simulink model "upqc"  (R2021a)
settings: Solver=VariableStepAuto  StartTime=0.0  StopTime=0.5  RelTol=1e-3
libraries: spsDiodeLib x18, spsSeriesRLCBranchLib x16, spsIGBTLib x6, spsCurrentMeasurementLib x5, spsGroundLib x3, spsThreePhaseSeriesRLCBranchLib x3, spsVoltageMeasurementLib x3, spsThreePhaseProgrammableVoltageSourceLib x3, spsThreePhaseVIMeasurementLib x3, spsPVArrayLib x1, spspowerguiLib x1
settings Model: Creator=Dell  LastModifiedBy=Dell

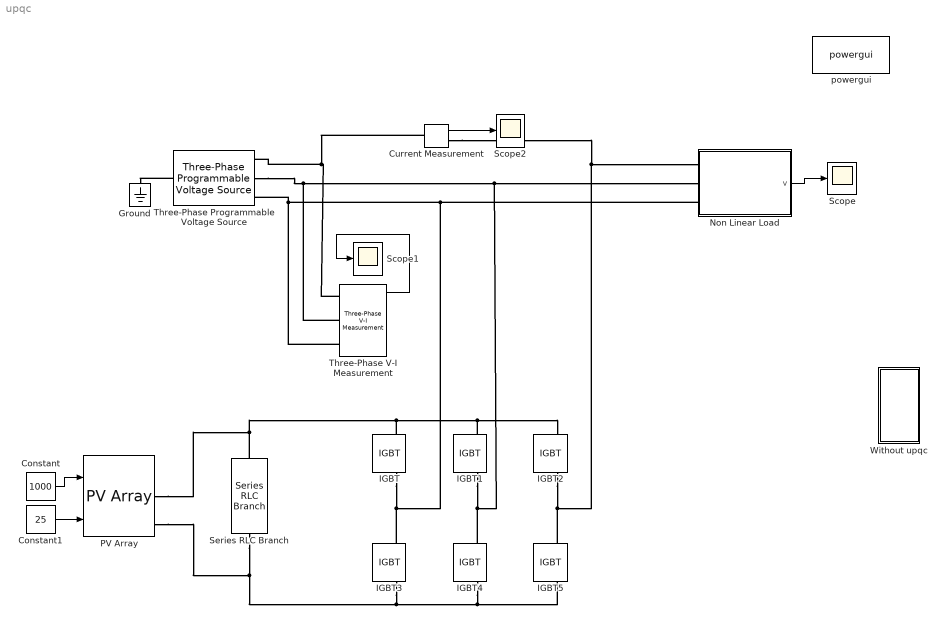
== system upqc ==
  Constant : Constant  Value=1000
  Constant1 : Constant  Value=25
  Current Measurement : spsCurrentMeasurementLib/Current Measurement  PhasorSimulation=off  OutputType=Complex  PSBequivalent=0
  Ground : spsGroundLib/Ground  LConnTagsString=a
  IGBT{,1..5} (6 alike) : spsIGBTLib/IGBT  Ron=0.001  Lon=0  Vf=1  Tf=1e-6  Tt=2e-6  IC=0  Rs=1e5  Cs=inf  Measurements=on
  Non Linear Load : Subsystem
  PV Array : spsPVArrayLib/PV Array  Npar=40  Nser=10  PlotType=array @ 1000 W/m2 & specified temperatures  S_vec="[ 1000  500  100 ]"  Temp_C_vec="[ 45 25  ]"  ModuleName=User-defined  PlotWhenSelected=off  Pm=213.15  Ncell=60  Voc=36.3  Isc=7.84  Vm=29  Im=7.35  beta_Voc_pc=-0.36099  alpha_Isc_pc=0.102  beta_Voc=-0.13104  alpha_Isc=0.0079968  IL=7.8654  I0=2.9273e-10  nI=0.98119  Rsh=313.0553  Rs=0.39381  RobustModel=off  RobustCellTemperature=313.3991  BAL=on  Tc=1e-6  Tfilter=5e-5
  Scope : Scope
  Scope1 : Scope
  Scope2 : Scope
  Series RLC Branch : spsSeriesRLCBranchLib/Series RLC Branch  LConnTagsString=__new0  RConnTagsString=__new0  BranchType=C  Resistance=1  Inductance=1e-3  SetiL0=off  InitialCurrent=0  Capacitance=1e-6  Setx0=off  InitialVoltage=0  Measurements=None
  Three-Phase Programmable Voltage Source : spsThreePhaseProgrammableVoltageSourceLib/Three-Phase Programmable Voltage Source  PositiveSequence="[400  0 50]"  VariationEntity=Amplitude  VariationType=Table of time-amplitude pairs  VariationTypeAlt=Step  VariationStep=0.5  VariationRate=10  VariationMagnitude=0.3  VariationFrequency=2  VariationTiming=[1 2]  VariationPhaseA=off  Amplitudes=[1 0.7 1 1.3 1]  TimeValues=[0 0.9 1 1.6 1.7]  HarmonicGeneration=on  HarmonicA=[5 0.2 -0 2]  HarmonicB=[7 0.05 0 1]  Timing=[0.3 0.4]  BusType=swing  Pref=0  Qref=0  Qmin=-inf  Qmax=inf
  Three-Phase V-I Measurement : spsThreePhaseVIMeasurementLib/Three-Phase V-I Measurement  VoltageMeasurement=phase-to-ground  SetLabelV=off  LabelV=Vabc  Vpu=off  VpuLL=off  CurrentMeasurement=yes  SetLabelI=off  LabelI=Iabc  Ipu=off  Pbase=100e6  Vbase=500e3  OutputType=Complex  PhasorSimulation=off  PSBequivalent=0
  Without upqc : Subsystem
  powergui : spspowerguiLib/powergui  Priority=1  SimulationMode=Continuous  SampleTime=50e-6  frequency=60  Iterations=50  frequencyindice=50  Pbase=100e6  ErrMax=1e-4  UnitsV=kV  UnitsW=MW  buscounter=0  FunctionMessages=off  echomessages=off  EnableUseOfTLC=off  CurrentSourceSwitches=off  DisableSnubberDevices=off  DisableRonSwitches=off  DisableVfSwitches=off  DisplayEquations=off  AutomaticDiscreteSolvers=off  SolverType=Tustin/Backward Euler (TBE)  Interpol=off  ExternalGateDelay=off  methode=off  Ts=100  x0status=blocks  SPID=on  SwTol=0  HookPort=off  NonlinearTolerance=1e-4  nMaxIteration=100  ContinueOnMaxIteration=off  RestoreLinks=warning  ResistiveCurrentMeasurement=off  Frange=[0:2:500]  Ylog=off  Xlog=on  ShowGrid=off  save=off  variable=ZData  structure=0  ZoomFFT=off  StartTime=0.0  cycles=1  DisplayStyle=1  fundamental=60  FreqAxis=off  MaxFrequency=1000  frequencyindicesteady=1  RmsSteady=1  display=off
  wires:
  Three-Phase V-I Measurement/1 -> Scope1/1
  Non Linear Load/1(v) -> Scope/1
  Constant1/1 -> PV Array/2
  Constant/1 -> PV Array/1
  Current Measurement/1 -> Scope2/1
  connections:
  Three-Phase Programmable Voltage Source/LConn1 -- Ground/LConn1
  Three-Phase V-I Measurement/LConn3 -- IGBT/RConn1 -- IGBT3/LConn1 -- Non Linear Load/LConn3 -- Three-Phase Programmable Voltage Source/RConn3
  Three-Phase V-I Measurement/LConn2 -- Three-Phase Programmable Voltage Source/RConn2 -- IGBT1/RConn1 -- IGBT4/LConn1 -- Non Linear Load/LConn2
  IGBT5/LConn1 -- IGBT2/RConn1 -- Current Measurement/RConn1 -- Non Linear Load/LConn1
  IGBT/LConn1 -- PV Array/RConn1 -- Series RLC Branch/LConn1 -- IGBT1/LConn1 -- IGBT2/LConn1
  IGBT3/RConn1 -- Series RLC Branch/RConn1 -- PV Array/RConn2 -- IGBT4/RConn1 -- IGBT5/RConn1
  Three-Phase V-I Measurement/LConn1 -- Current Measurement/LConn1 -- Three-Phase Programmable Voltage Source/RConn1

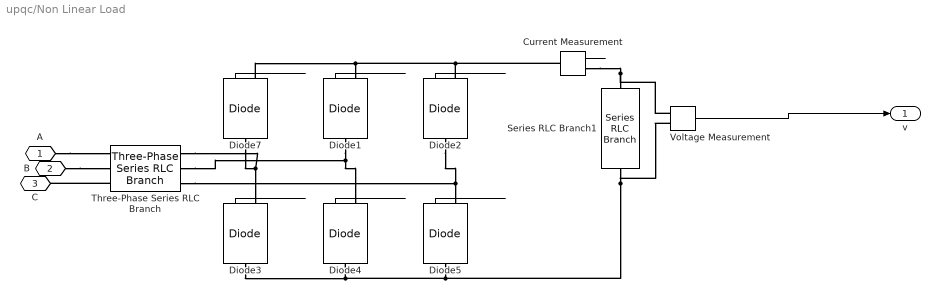
== system upqc/Non Linear Load ==
  Current Measurement : spsCurrentMeasurementLib/Current Measurement  PhasorSimulation=off  OutputType=Complex  PSBequivalent=0
  Diode{1..5,7} (6 alike) : spsDiodeLib/Diode  Ron=0.001  Lon=0  Vf=0.8  IC=0  UseSnubber=0  Rs=500  Cs=250e-9  Measurements=on
  Series RLC Branch1 : spsSeriesRLCBranchLib/Series RLC Branch  LConnTagsString=__new0  RConnTagsString=__new0  BranchType=RL  Resistance=1  Inductance=1e-3  SetiL0=off  InitialCurrent=0  Capacitance=1e-6  Setx0=off  InitialVoltage=0  Measurements=None
  Three-Phase Series RLC Branch : spsThreePhaseSeriesRLCBranchLib/Three-Phase Series RLC Branch  LConnTagsString=A|B|C  RConnTagsString=A|B|C  BranchType=RL  Resistance=1  Inductance=1e-3  Capacitance=1e-6  Measurements=None
  Voltage Measurement : spsVoltageMeasurementLib/Voltage Measurement  PhasorSimulation=off  OutputType=Complex  PSBequivalent=0
  A : PMIOPort  Side=Left
  B : PMIOPort  Port=2  Side=Left
  C : PMIOPort  Port=3  Side=Left
  v : Outport
  wires:
  Diode5/1 -> ?
  Diode2/1 -> ?
  Current Measurement/1 -> ?
  Diode1/1 -> ?
  Diode7/1 -> ?
  Voltage Measurement/1 -> v/1
  Diode4/1 -> ?
  Diode3/1 -> ?
  connections:
  Diode2/LConn1 -- Diode5/RConn1 -- Three-Phase Series RLC Branch/RConn3
  Diode3/LConn1 -- Voltage Measurement/LConn2 -- Series RLC Branch1/RConn1 -- Diode5/LConn1 -- Diode4/LConn1
  Diode1/LConn1 -- Diode4/RConn1 -- Three-Phase Series RLC Branch/RConn2
  Current Measurement/RConn1 -- Voltage Measurement/LConn1 -- Series RLC Branch1/LConn1
  Diode7/RConn1 -- Current Measurement/LConn1 -- Diode2/RConn1 -- Diode1/RConn1
  Diode7/LConn1 -- Diode3/RConn1 -- Three-Phase Series RLC Branch/RConn1
  Three-Phase Series RLC Branch/LConn3 -- C/RConn1
  A/RConn1 -- Three-Phase Series RLC Branch/LConn1
  B/RConn1 -- Three-Phase Series RLC Branch/LConn2

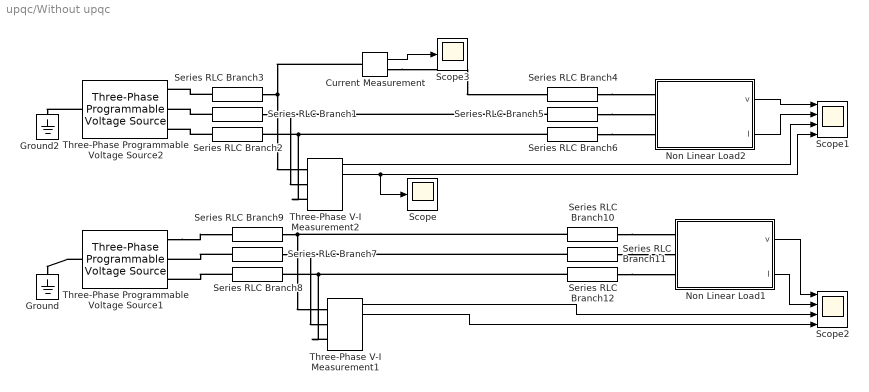
== system upqc/Without upqc ==
  Current Measurement : spsCurrentMeasurementLib/Current Measurement  PhasorSimulation=off  OutputType=Complex  PSBequivalent=0
  Ground : spsGroundLib/Ground  LConnTagsString=a
  Ground2 : spsGroundLib/Ground  LConnTagsString=a
  Non Linear Load1 : Subsystem
  Non Linear Load2 : Subsystem
  Scope : Scope
  Scope1 : Scope  NumInputPorts=4
  Scope2 : Scope  NumInputPorts=4
  Scope3 : Scope
  Series RLC Branch{1..12} (12 alike) : spsSeriesRLCBranchLib/Series RLC Branch  LConnTagsString=__new0  RConnTagsString=__new0  BranchType=RL  Resistance=2000  Inductance=1e-3  SetiL0=off  InitialCurrent=0  Capacitance=1e-6  Setx0=off  InitialVoltage=0  Measurements=None
  Three-Phase Programmable Voltage Source1 : spsThreePhaseProgrammableVoltageSourceLib/Three-Phase Programmable Voltage Source  PositiveSequence="[400  0 50]"  VariationEntity=Amplitude  VariationType=Table of time-amplitude pairs  VariationTypeAlt=Step  VariationStep=0.5  VariationRate=10  VariationMagnitude=0.3  VariationFrequency=2  VariationTiming=[1 2]  VariationPhaseA=off  Amplitudes=[1 0.7 1 1.3 1]  TimeValues=[0 0.9 1 1.6 1.7]  HarmonicGeneration=on  HarmonicA=[5 0.2 -0 2]  HarmonicB=[7 0.05 0 1]  Timing=[0.3 0.4]  BusType=swing  Pref=0  Qref=0  Qmin=-inf  Qmax=inf
  Three-Phase Programmable Voltage Source2 : spsThreePhaseProgrammableVoltageSourceLib/Three-Phase Programmable Voltage Source  PositiveSequence="[400  0 50]"  VariationEntity=None  VariationType=Table of time-amplitude pairs  VariationTypeAlt=Step  VariationStep=0.5  VariationRate=10  VariationMagnitude=0.3  VariationFrequency=2  VariationTiming=[1 2]  VariationPhaseA=off  Amplitudes=[1 0.7 1 1.3 1]  TimeValues=[0 0.9 1 1.6 1.7]  HarmonicGeneration=off  HarmonicA=[5 0.2 -0 2]  HarmonicB=[7 0.05 0 1]  Timing=[0.3 0.4]  BusType=swing  Pref=0  Qref=0  Qmin=-inf  Qmax=inf
  Three-Phase V-I Measurement1 : spsThreePhaseVIMeasurementLib/Three-Phase V-I Measurement  VoltageMeasurement=phase-to-ground  SetLabelV=off  LabelV=Vabc  Vpu=off  VpuLL=off  CurrentMeasurement=yes  SetLabelI=off  LabelI=Iabc  Ipu=off  Pbase=100e6  Vbase=500e3  OutputType=Complex  PhasorSimulation=off  PSBequivalent=0
  Three-Phase V-I Measurement2 : spsThreePhaseVIMeasurementLib/Three-Phase V-I Measurement  VoltageMeasurement=phase-to-ground  SetLabelV=off  LabelV=Vabc  Vpu=off  VpuLL=off  CurrentMeasurement=yes  SetLabelI=off  LabelI=Iabc  Ipu=off  Pbase=100e6  Vbase=500e3  OutputType=Complex  PhasorSimulation=off  PSBequivalent=0
  wires:
  Non Linear Load2/1(v) -> Scope1/1
  Three-Phase V-I Measurement2/1 -> Scope1/3
  Non Linear Load2/2(I) -> Scope1/2
  Three-Phase V-I Measurement2/2 -> Scope/1, Scope1/4
  Three-Phase V-I Measurement1/2 -> Scope2/4
  Three-Phase V-I Measurement1/1 -> Scope2/3
  Non Linear Load1/2(I) -> Scope2/2
  Non Linear Load1/1(v) -> Scope2/1
  Current Measurement/1 -> Scope3/1
  connections:
  Series RLC Branch3/LConn1 -- Three-Phase Programmable Voltage Source2/RConn1
  Series RLC Branch1/LConn1 -- Three-Phase Programmable Voltage Source2/RConn2
  Series RLC Branch2/LConn1 -- Three-Phase Programmable Voltage Source2/RConn3
  Three-Phase Programmable Voltage Source2/LConn1 -- Ground2/LConn1
  Series RLC Branch3/RConn1 -- Current Measurement/LConn1 -- Three-Phase V-I Measurement2/LConn1
  Series RLC Branch1/RConn1 -- Series RLC Branch5/LConn1 -- Three-Phase V-I Measurement2/LConn2
  Three-Phase V-I Measurement2/LConn3 -- Series RLC Branch6/LConn1 -- Series RLC Branch2/RConn1
  Series RLC Branch4/RConn1 -- Non Linear Load2/LConn1
  Series RLC Branch5/RConn1 -- Non Linear Load2/LConn2
  Series RLC Branch6/RConn1 -- Non Linear Load2/LConn3
  Three-Phase V-I Measurement1/LConn3 -- Series RLC Branch12/LConn1 -- Series RLC Branch8/RConn1
  Series RLC Branch9/RConn1 -- Series RLC Branch10/LConn1 -- Three-Phase V-I Measurement1/LConn1
  Series RLC Branch7/RConn1 -- Series RLC Branch11/LConn1 -- Three-Phase V-I Measurement1/LConn2
  Series RLC Branch11/RConn1 -- Non Linear Load1/LConn2
  Series RLC Branch10/RConn1 -- Non Linear Load1/LConn1
  Series RLC Branch8/LConn1 -- Three-Phase Programmable Voltage Source1/RConn3
  Series RLC Branch7/LConn1 -- Three-Phase Programmable Voltage Source1/RConn2
  Series RLC Branch12/RConn1 -- Non Linear Load1/LConn3
  Three-Phase Programmable Voltage Source1/RConn1 -- Series RLC Branch9/LConn1
  Three-Phase Programmable Voltage Source1/LConn1 -- Ground/LConn1
  Current Measurement/RConn1 -- Series RLC Branch4/LConn1

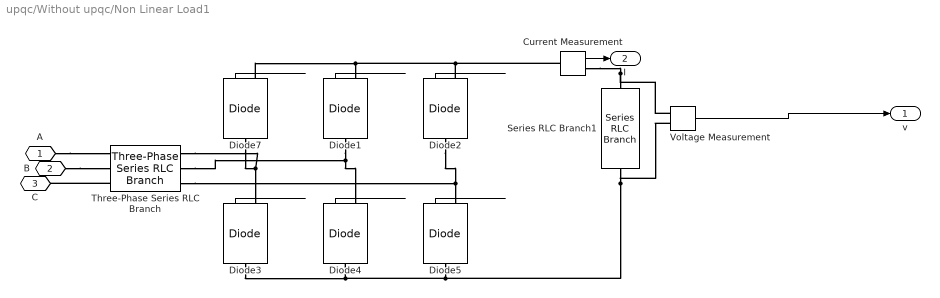
== system upqc/Without upqc/Non Linear Load1 ==
  Current Measurement : spsCurrentMeasurementLib/Current Measurement  PhasorSimulation=off  OutputType=Complex  PSBequivalent=0
  Diode{1..5,7} (6 alike) : spsDiodeLib/Diode  Ron=0.001  Lon=0  Vf=0.8  IC=0  UseSnubber=0  Rs=500  Cs=250e-9  Measurements=on
  Series RLC Branch1 : spsSeriesRLCBranchLib/Series RLC Branch  LConnTagsString=__new0  RConnTagsString=__new0  BranchType=RL  Resistance=1  Inductance=1e-3  SetiL0=off  InitialCurrent=0  Capacitance=1e-6  Setx0=off  InitialVoltage=0  Measurements=None
  Three-Phase Series RLC Branch : spsThreePhaseSeriesRLCBranchLib/Three-Phase Series RLC Branch  LConnTagsString=A|B|C  RConnTagsString=A|B|C  BranchType=RL  Resistance=1  Inductance=1e-3  Capacitance=1e-6  Measurements=None
  Voltage Measurement : spsVoltageMeasurementLib/Voltage Measurement  PhasorSimulation=off  OutputType=Complex  PSBequivalent=0
  A : PMIOPort  Side=Left
  B : PMIOPort  Port=2  Side=Left
  C : PMIOPort  Port=3  Side=Left
  v : Outport
  I : Outport  Port=2
  wires:
  Diode5/1 -> ?
  Diode2/1 -> ?
  Current Measurement/1 -> I/1
  Diode1/1 -> ?
  Diode7/1 -> ?
  Voltage Measurement/1 -> v/1
  Diode4/1 -> ?
  Diode3/1 -> ?
  connections:
  Diode2/LConn1 -- Diode5/RConn1 -- Three-Phase Series RLC Branch/RConn3
  Diode3/LConn1 -- Voltage Measurement/LConn2 -- Series RLC Branch1/RConn1 -- Diode5/LConn1 -- Diode4/LConn1
  Diode1/LConn1 -- Diode4/RConn1 -- Three-Phase Series RLC Branch/RConn2
  Current Measurement/RConn1 -- Voltage Measurement/LConn1 -- Series RLC Branch1/LConn1
  Diode7/RConn1 -- Current Measurement/LConn1 -- Diode2/RConn1 -- Diode1/RConn1
  Diode7/LConn1 -- Diode3/RConn1 -- Three-Phase Series RLC Branch/RConn1
  Three-Phase Series RLC Branch/LConn3 -- C/RConn1
  A/RConn1 -- Three-Phase Series RLC Branch/LConn1
  B/RConn1 -- Three-Phase Series RLC Branch/LConn2

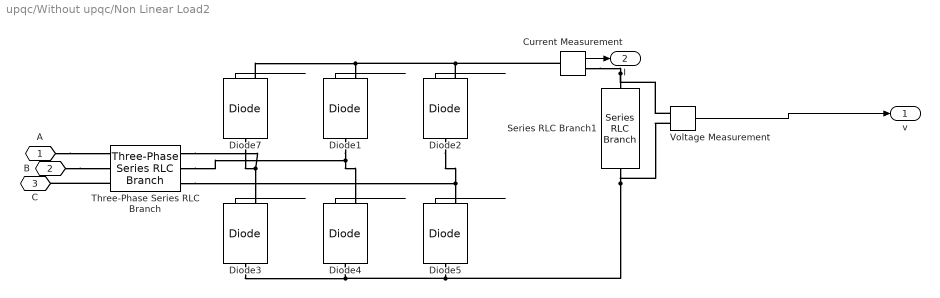
== system upqc/Without upqc/Non Linear Load2 ==
  Current Measurement : spsCurrentMeasurementLib/Current Measurement  PhasorSimulation=off  OutputType=Complex  PSBequivalent=0
  Diode{1..5,7} (6 alike) : spsDiodeLib/Diode  Ron=0.001  Lon=0  Vf=0.8  IC=0  UseSnubber=0  Rs=500  Cs=250e-9  Measurements=on
  Series RLC Branch1 : spsSeriesRLCBranchLib/Series RLC Branch  LConnTagsString=__new0  RConnTagsString=__new0  BranchType=RL  Resistance=1  Inductance=1e-3  SetiL0=off  InitialCurrent=0  Capacitance=1e-6  Setx0=off  InitialVoltage=0  Measurements=None
  Three-Phase Series RLC Branch : spsThreePhaseSeriesRLCBranchLib/Three-Phase Series RLC Branch  LConnTagsString=A|B|C  RConnTagsString=A|B|C  BranchType=RL  Resistance=1  Inductance=1e-3  Capacitance=1e-6  Measurements=None
  Voltage Measurement : spsVoltageMeasurementLib/Voltage Measurement  PhasorSimulation=off  OutputType=Complex  PSBequivalent=0
  A : PMIOPort  Side=Left
  B : PMIOPort  Port=2  Side=Left
  C : PMIOPort  Port=3  Side=Left
  v : Outport
  I : Outport  Port=2
  wires:
  Diode5/1 -> ?
  Diode2/1 -> ?
  Current Measurement/1 -> I/1
  Diode1/1 -> ?
  Diode7/1 -> ?
  Voltage Measurement/1 -> v/1
  Diode4/1 -> ?
  Diode3/1 -> ?
  connections:
  Diode2/LConn1 -- Diode5/RConn1 -- Three-Phase Series RLC Branch/RConn3
  Diode3/LConn1 -- Voltage Measurement/LConn2 -- Series RLC Branch1/RConn1 -- Diode5/LConn1 -- Diode4/LConn1
  Diode1/LConn1 -- Diode4/RConn1 -- Three-Phase Series RLC Branch/RConn2
  Current Measurement/RConn1 -- Voltage Measurement/LConn1 -- Series RLC Branch1/LConn1
  Diode7/RConn1 -- Current Measurement/LConn1 -- Diode2/RConn1 -- Diode1/RConn1
  Diode7/LConn1 -- Diode3/RConn1 -- Three-Phase Series RLC Branch/RConn1
  Three-Phase Series RLC Branch/LConn3 -- C/RConn1
  A/RConn1 -- Three-Phase Series RLC Branch/LConn1
  B/RConn1 -- Three-Phase Series RLC Branch/LConn2
